simulink model "FILE3_s_2dof_Model_vis"  (R2021b)
settings: Solver=VariableStepAuto  StartTime=0.0  StopTime=10.0  MaxStep=1e-3  RelTol=1e-3
libraries: simulink_extras x2
settings Model: Creator=artur  LastModifiedBy=artur

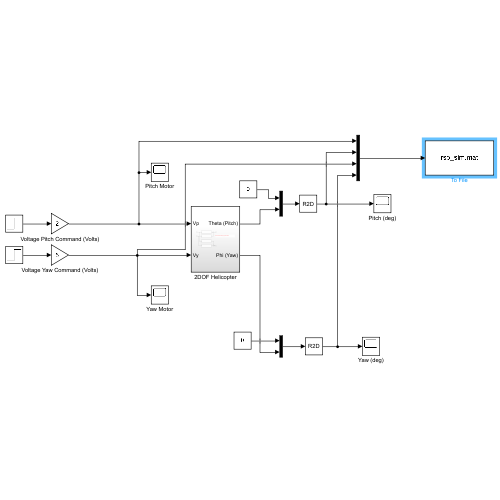
[thumbnail: Simulink's stored preview of the top-level diagram]
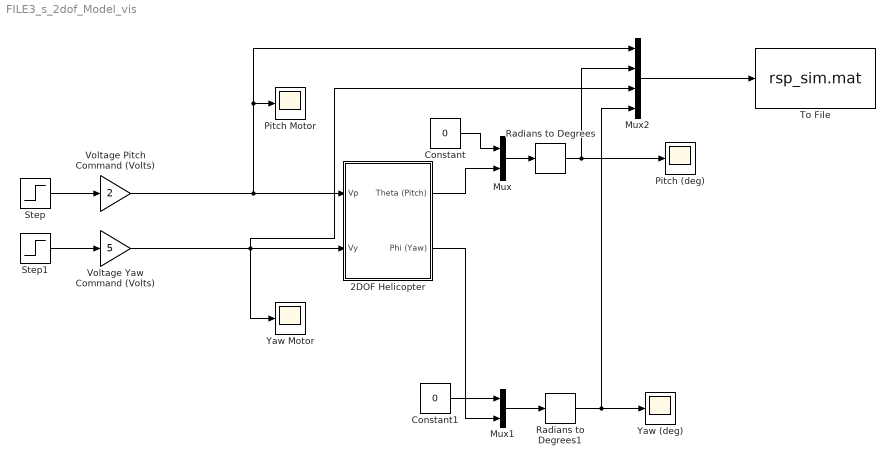
== system FILE3_s_2dof_Model_vis ==
  2DOF Helicopter : Subsystem
  Constant : Constant  Value=0
  Constant1 : Constant  Value=0
  Mux : Mux  Inputs=2
  Mux1 : Mux  Inputs=2
  Mux2 : Mux
  Pitch (deg) : Scope
  Pitch Motor : Scope
  Radians to Degrees : simulink_extras/Transformations/Radians to Degrees
  Radians to Degrees1 : simulink_extras/Transformations/Radians to Degrees
  Step : Step  SampleTime=0
  Step1 : Step  SampleTime=0
  To File : ToFile  Filename=rsp_sim.mat  MatrixName=rsp_sim
  Voltage Pitch Command (Volts) : Gain  Gain=2
  Voltage Yaw Command (Volts) : Gain  Gain=5
  Yaw (deg) : Scope
  Yaw Motor : Scope
  wires:
  Constant1/1 -> Mux1/1
  Radians to Degrees1/1 -> Mux2/4, Yaw (deg)/1
  Mux1/1 -> Radians to Degrees1/1
  Step1/1 -> Voltage Yaw Command (Volts)/1
  Radians to Degrees/1 -> Pitch (deg)/1, Mux2/2
  Voltage Yaw Command (Volts)/1 -> Yaw Motor/1, 2DOF Helicopter/2(Vy), Mux2/3
  Constant/1 -> Mux/1
  Mux2/1 -> To File/1
  Voltage Pitch Command (Volts)/1 -> Pitch Motor/1, Mux2/1, 2DOF Helicopter/1(Vp)
  2DOF Helicopter/1(Theta (Pitch)) -> Mux/2
  Step/1 -> Voltage Pitch Command (Volts)/1
  2DOF Helicopter/2(Phi (Yaw)) -> Mux1/2
  Mux/1 -> Radians to Degrees/1

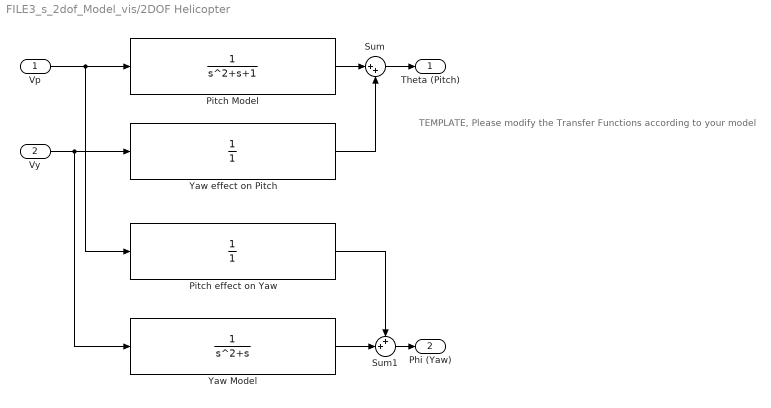
== system FILE3_s_2dof_Model_vis/2DOF Helicopter ==
  note: TEMPLATE, Please modify the Transfer Functions according to your model
  Vp : Inport
  Vy : Inport  Port=2
  Pitch Model : TransferFcn  Denominator=[1 1 1]
  Pitch effect on Yaw : TransferFcn  Denominator=[1]
  Sum : Sum  Inputs=|++
  Sum1 : Sum  Inputs=++|
  Yaw Model : TransferFcn  Denominator=[1 1 0]
  Yaw effect on Pitch : TransferFcn  Denominator=[1]
  Theta (Pitch) : Outport
  Phi (Yaw) : Outport  Port=2
  wires:
  Vp/1 -> Pitch effect on Yaw/1, Pitch Model/1
  Vy/1 -> Yaw Model/1, Yaw effect on Pitch/1
  Pitch Model/1 -> Sum/1
  Sum/1 -> Theta (Pitch)/1
  Yaw effect on Pitch/1 -> Sum/2
  Sum1/1 -> Phi (Yaw)/1
  Yaw Model/1 -> Sum1/2
  Pitch effect on Yaw/1 -> Sum1/1
